simulink library "BUS_Time_Bus_Reset"  (R2018b)
settings: Solver=VariableStepAuto  StartTime=0.0  StopTime=10.0  RelTol=1e-3
settings Model: Creator=Alexander Koch  LastModifiedBy=ga69qig
settings SFSimCC: SimUseLocalCustomCode=off
settings RTWCC: RTWUseLocalCustomCode=off
settings CodeAppCC: StateflowObjectComments=on

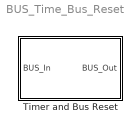
== system BUS_Time_Bus_Reset ==
  Timer and Bus Reset : Subsystem
      mask help:
      | <Author> Alexander Koch based on Stefan Müller, Stephan Rohr
      | <Date> 03/04/2017
      |
      | <Description>
      | Initiate a new timestep and creates the Bus_Old with all data of the last time step
      settings: OpenFcn=|
      | set_param(gcb(),'LinkStatus','none')
      | open_system(gcb(),'mask')
      mask DialogControl RefreshBus Prompt: Refresh Bus
      mask DialogControl RefreshBus Callback: TimerandBusResetRefreshBus()

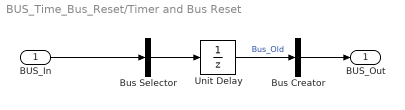
== system BUS_Time_Bus_Reset/Timer and Bus Reset ==
  BUS_In : Inport
  Bus Creator : BusCreator  Inputs=1
  Bus Selector : BusSelector  OutputSignals=signal1  OutputAsBus=on
  Unit Delay : UnitDelay  SampleTime=-1
  BUS_Out : Outport
  wires:
  BUS_In/1 -> Bus Selector/1
  Unit Delay/1 -> Bus Creator/1  "Bus_Old"
  Bus Selector/1 -> Unit Delay/1
  Bus Creator/1 -> BUS_Out/1
